simulink model "three_link_inverse_control"  (R2021b)
settings: Solver=FixedStepAuto  StartTime=0.0  StopTime=10  FixedStep=0.01  RelTol=1e-3
InitFcn:
  | stop_time_as_str = get_param(gcs, 'StopTime');
  | stopTime = str2double(stop_time_as_str);
values from neighbouring files (symbols this model uses):
  q1 = UnitQuaternion(R)    [Basiccommands_for_representing_position_and_orientation.m]
  q2 = q1.inv    [Basiccommands_for_representing_position_and_orientation.m]
undefined symbols (not defined in the file or in its folder): g, KD, KP, max_torques, min_torques, q3, qdot1, qdot2, qdot3, subs, vB, vC, vF, vG
libraries: roblocks x3
settings Model: Creator=jan  LastModifiedBy=Ilyass
settings SolverCC: AlgebraicLoopSolver=TrustRegion
settings DataIOCC: ReturnWorkspaceOutputs=off
settings DebuggingCC: SFMachineParentedDataDiag=warning  ArithmeticOperatorsInVariantConditions=warning
settings SFSimCC: SimUseLocalCustomCode=off  CustomCodeUndefinedFunction=UseInterfaceOnly
settings RTWCC: RTWUseLocalCustomCode=off

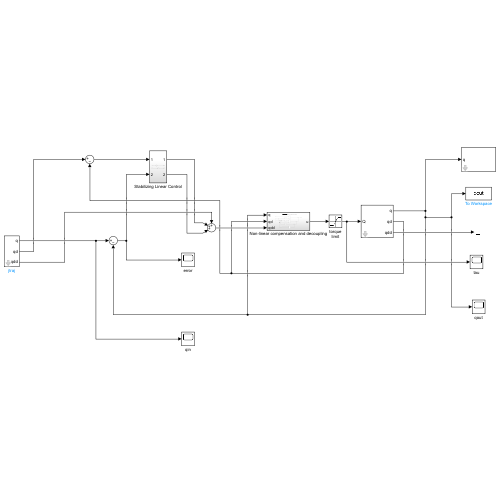
[thumbnail: Simulink's stored preview of the top-level diagram]
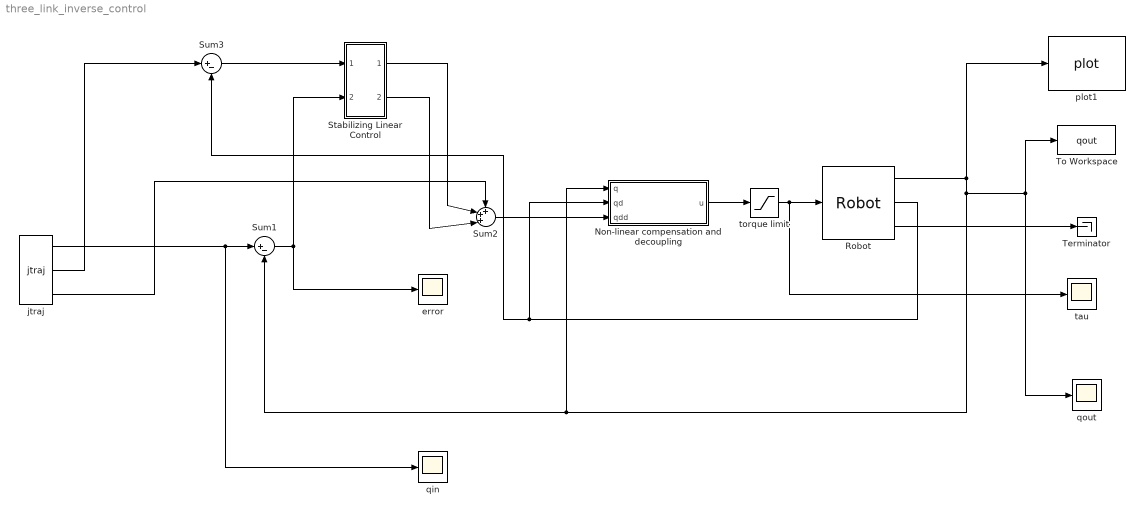
== system three_link_inverse_control ==
  Non-linear compensation and decoupling : Subsystem
  Robot : roblocks/Arm/Robot  robot=threelink  q0=[0 0 0]
  Stabilizing Linear Control : Subsystem
  Sum1 : Sum  Inputs=|+-
  Sum2 : Sum  Inputs=+++|
  Sum3 : Sum  Inputs=|+-
  Terminator : Terminator
  To Workspace : ToWorkspace  VariableName=qout  SaveFormat=Timeseries  SampleTime=-1
  error : Scope
  jtraj : roblocks/Toolbox/jtraj  q0=[0 0 0]  qf=[pi/4 pi/4 pi/4]  tmax=stopTime  ts=0.02
  plot1 : roblocks/Arm/plot  robot=threelink  fps=20  holdplot=off
  qin : Scope
  qout : Scope
  tau : Scope
  torque limit : Saturate  UpperLimit=max_torques  LowerLimit=min_torques
  wires:
  Robot/3 -> Terminator/1
  Sum1/1 -> Stabilizing Linear Control/2(In2), error/1
  jtraj/1 -> qin/1, Sum1/1
  torque limit/1 -> Robot/1, tau/1
  Sum2/1 -> Non-linear compensation and decoupling/3(qdd)
  jtraj/3 -> Sum2/1
  jtraj/2 -> Sum3/1
  Non-linear compensation and decoupling/1(u) -> torque limit/1
  Sum3/1 -> Stabilizing Linear Control/1(In1)
  Stabilizing Linear Control/1(Out1) -> Sum2/2
  Stabilizing Linear Control/2(Out2) -> Sum2/3
  Robot/1 -> Non-linear compensation and decoupling/1(q), Sum1/2, To Workspace/1, qout/1, plot1/1
  Robot/2 -> Non-linear compensation and decoupling/2(qd), Sum3/2

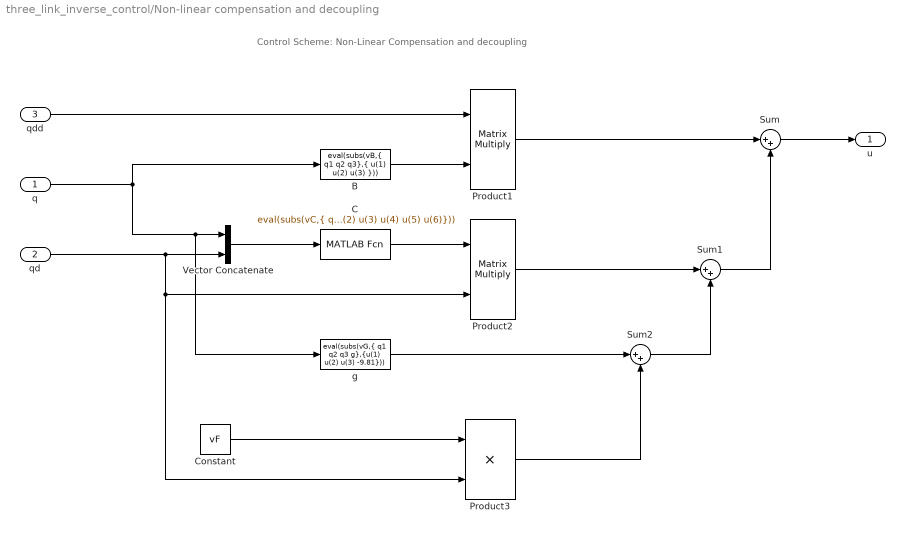
== system three_link_inverse_control/Non-linear compensation and decoupling ==
  note: Control Scheme: Non-Linear Compensation and decoupling
  q : Inport
  qd : Inport  Port=2
  qdd : Inport  Port=3
  B : MATLABFcn  MATLABFcn=eval(subs(vB,{ q1 q2 q3},{ u(1) u(2) u(3) }))  OutputDimensions=[3 3]  Output1D=off
  C : MATLABFcn  MATLABFcn=eval(subs(vC,{ q1 q2 q3 qdot1 qdot2 qdot3 },{ u(1) u(2) u(3) u(4) u(5) u(6)}))  OutputDimensions=[3 3]  Output1D=off
  Constant : Constant  Value=vF
  Product1 : Product  Multiplication=Matrix(*)  RndMeth=Zero
  Product2 : Product  Multiplication=Matrix(*)  RndMeth=Zero
  Product3 : Product  RndMeth=Zero
  Sum : Sum  Inputs=|++
  Sum1 : Sum  Inputs=|++
  Sum2 : Sum  Inputs=|++
  Vector Concatenate : Concatenate
  g : MATLABFcn  MATLABFcn=eval(subs(vG,{ q1 q2 q3 g},{u(1) u(2) u(3) -9.81}))  OutputDimensions=[1 3]  Output1D=off
  u : Outport  VectorParamsAs1DForOutWhenUnconnected=off
  wires:
  q/1 -> B/1, g/1, Vector Concatenate/1
  qd/1 -> Product3/2, Product2/2, Vector Concatenate/2
  qdd/1 -> Product1/1
  B/1 -> Product1/2
  Vector Concatenate/1 -> C/1
  C/1 -> Product2/1
  Product1/1 -> Sum/1
  Sum/1 -> u/1
  Product2/1 -> Sum1/1
  Sum1/1 -> Sum/2
  Constant/1 -> Product3/1
  g/1 -> Sum2/1
  Product3/1 -> Sum2/2
  Sum2/1 -> Sum1/2

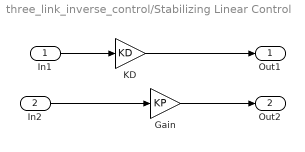
== system three_link_inverse_control/Stabilizing Linear Control ==
  In1 : Inport
  In2 : Inport  Port=2
  Gain : Gain  Gain=KP
  KD : Gain  Gain=KD
  Out1 : Outport
  Out2 : Outport  Port=2
  wires:
  In2/1 -> Gain/1
  In1/1 -> KD/1
  Gain/1 -> Out2/1
  KD/1 -> Out1/1
